simulink model "testFrame_PositionObserever"  (R2020b)
settings: Solver=FixedStepDiscrete  StartTime=0.0  StopTime=100  FixedStep=50e-6  RelTol=1e-3
undefined symbols (not defined in the file): d_q_Voltage_Limiter_sat_neg, d_q_Voltage_Limiter_sat_pos, Ts
libraries: mcbcontrolslib x4, pid_lib x2, simulink x1
settings Model: DataDictionary=MotorControl.sldd  NumberOfSteps=10  Creator=unix  LastModifiedBy=unix
settings DebuggingCC: IntegerOverflowMsg=error  ParameterUnderflowMsg=error  IntegerSaturationMsg=error

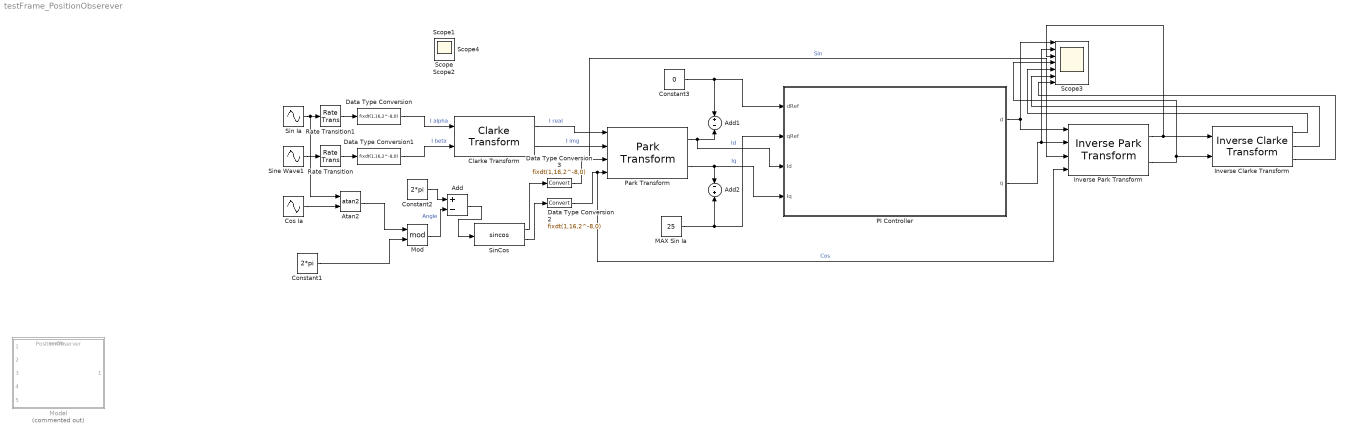
== system testFrame_PositionObserever ==
  Add : Sum  Inputs=+-
  Add1 : Sum  Inputs=+-  OutDataTypeStr=Inherit: Inherit via back propagation
  Add2 : Sum  Inputs=-+
  Atan2 : Trigonometry  Operator=atan2
  Clarke Transform : mcbcontrolslib/Clarke Transform  VariantControl=Variant2
  Constant1 : Constant  Value=2*pi  OutDataTypeStr=Inherit: Inherit via back propagation
  Constant2 : Constant  Value=2*pi  OutDataTypeStr=Inherit: Inherit via back propagation
  Constant3 : Constant  Value=0  OutDataTypeStr=int8
  Cos Ia : Sin  Amplitude=25  Frequency=100  Phase=pi/2  SampleTime=0
  Data Type Conversion{,1..3} (4 alike) : DataTypeConversion  OutDataTypeStr=fixdt(1,16,2^-8,0)
  Inverse Clarke Transform : mcbcontrolslib/Inverse Clarke Transform
      settings: SourceProductBaseCode=MT
  Inverse Park Transform : mcbcontrolslib/Inverse Park Transform  AxisAlignment=D-axis
  MAX Sin Ia : Constant  Value=25  OutDataTypeStr=Inherit: Inherit via back propagation
  Mod : Math  Operator=mod  SaturateOnIntegerOverflow=on
  Model : ModelReference  Commented=on  ModelNameDialog=PositionObserver.slx  ModelReferenceVersion=3.3  EnablePortName=Enable  EnablePortStatesWhenEnabling=reset
  PI Controller : Subsystem
  Park Transform : mcbcontrolslib/Park Transform  AxisAlignment=D-axis
      settings: SourceProductBaseCode=MT
  Rate Transition : RateTransition  OutPortSampleTime=250e-6
  Rate Transition1 : RateTransition  OutPortSampleTime=250e-6
  Scope3 : Scope  NumInputPorts=7
  Sin Ia : Sin  Amplitude=25  Frequency=100  SampleTime=0
  SinCos : Trigonometry  Operator=sincos
  Sine Wave1 : Sin  Amplitude=25  Frequency=100  Phase=(2*pi)/3  SampleTime=0
  Scope{,1..2,4} (4 alike) : Scope
  wires:
  SinCos/2 -> Data Type Conversion2/1
  SinCos/1 -> Data Type Conversion3/1
  Sin Ia/1 -> Atan2/1, Rate Transition1/1
  Sine Wave1/1 -> Rate Transition/1
  Clarke Transform/1 -> Park Transform/1  "I real"
  Clarke Transform/2 -> Park Transform/2  "I img"
  Constant1/1 -> Mod/2
  Park Transform/1 -> Add1/2, PI Controller/3(Id)  "Id"
  Park Transform/2 -> Add2/1, PI Controller/4(Iq)  "Iq"
  Data Type Conversion/1 -> Clarke Transform/1  "I alpha"
  Data Type Conversion1/1 -> Clarke Transform/2  "I beta"
  Mod/1 -> Add/2  "Angle"
  Data Type Conversion2/1 -> Inverse Park Transform/4, Park Transform/4  "Cos"
  Data Type Conversion3/1 -> Inverse Park Transform/3, Park Transform/3  "Sin"
  Rate Transition/1 -> Data Type Conversion1/1
  Rate Transition1/1 -> Data Type Conversion/1
  Constant2/1 -> Add/1
  Add/1 -> SinCos/1
  Constant3/1 -> Add1/1, PI Controller/1(dRef)
  MAX Sin Ia/1 -> Add2/2, PI Controller/2(qRef)
  PI Controller/1(d) -> Inverse Park Transform/1, Scope3/1
  PI Controller/2(q) -> Inverse Park Transform/2, Scope3/2
  Cos Ia/1 -> Atan2/2
  Atan2/1 -> Mod/1
  Inverse Park Transform/1 -> Inverse Clarke Transform/1, Scope3/3
  Inverse Park Transform/2 -> Inverse Clarke Transform/2, Scope3/4
  Inverse Clarke Transform/1 -> Scope3/5
  Inverse Clarke Transform/2 -> Scope3/6
  Inverse Clarke Transform/3 -> Scope3/7

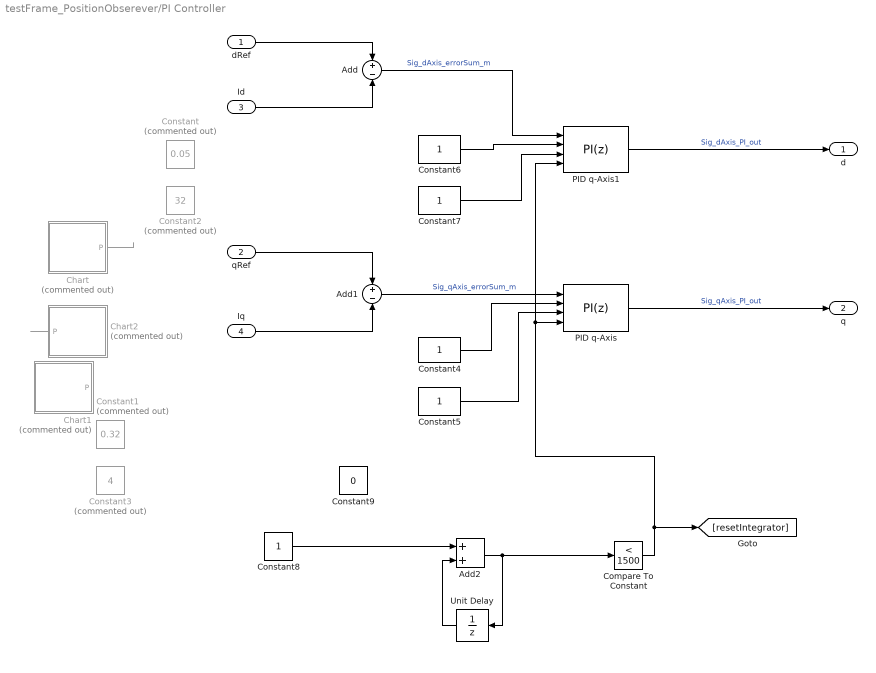
== system testFrame_PositionObserever/PI Controller ==
  dRef : Inport
  qRef : Inport  Port=2
  Id : Inport  Port=3
  Iq : Inport  Port=4
  Add : Sum  Inputs=+|-
  Add1 : Sum  Inputs=+|-
  Add2 : Sum
  Chart : Stateflow chart  Commented=on  TreatAsAtomicUnit=on  SystemSampleTime=1000*Ts
  Chart1 : Stateflow chart  Commented=on  TreatAsAtomicUnit=on  SystemSampleTime=2000*Ts
  Chart2 : Stateflow chart  Commented=on  TreatAsAtomicUnit=on  SystemSampleTime=100000*Ts
  Compare To Constant : simulink/Logic and Bit Operations/Compare To Constant  relop=<  const=1500  OutDataTypeStr=boolean
  Constant : Constant  Commented=on  Value=0.05  OutDataTypeStr=fixdt(1,16,2^-7,0)
  Constant1 : Constant  Commented=on  Value=0.32  OutDataTypeStr=fixdt(1,8,2^-7,0)
  Constant2 : Constant  Commented=on  Value=32  OutDataTypeStr=fixdt(1,8,2^-1,0)
  Constant3 : Constant  Commented=on  Value=4  OutDataTypeStr=fixdt(1,8,2^-1,0)
  Constant{4..7} (4 alike) : Constant  OutDataTypeStr=fixdt(1,16,2^-5,0)
  Constant8 : Constant
  Constant9 : Constant  Value=0  OutDataTypeStr=boolean
  PID q-Axis : pid_lib/PID Controller  Controller=PI  Form=Parallel  TimeDomain=Discrete-time  UseExternalTs=off  SampleTime=-1  IntegratorMethod=Forward Euler  FilterMethod=Forward Euler  ControllerParametersSource=external  P=0  I=0  D=0  UseFilter=on  N=100  TunerSelectOption=Transfer Function Based (PID Tuner App)  InitialConditionSource=internal  InitialConditionForIntegrator=0  InitialConditionForFilter=0  DifferentiatorICPrevScaledInput=0  ExternalReset=level  TrackingMode=off  Kt=1  LimitOutput=on  SatLimitsSource=internal  UpperSaturationLimit=d_q_Voltage_Limiter_sat_pos  LowerSaturationLimit=d_q_Voltage_Limiter_sat_neg  LinearizeAsGain=off  AntiWindupMode=clamping  Kb=10  PGainOutDataTypeStr=fixdt(1,16,2^-8,0)  PProdOutDataTypeStr=fixdt(1,16,2^-8,0)  POutMin=[]  POutMax=[]  IGainOutDataTypeStr=fixdt(1,16,2^-8,0)  IProdOutDataTypeStr=fixdt(1,16,2^-8,0)  IOutMin=[]  IOutMax=[]  DOutMin=[]  DOutMax=[]  NOutMin=[]  NOutMax=[]  SumOutDataTypeStr=fixdt(1,16,2^-8,0)  SumOutMin=[]  SumOutMax=[]  SaturationOutMin=[]  SaturationOutMax=[]  PParamMin=[]  PParamMax=[]  IParamMin=[]  IParamMax=[]  DParamMin=[]  DParamMax=[]  NParamMin=[]  NParamMax=[]  KbParamMin=[]  KbParamMax=[]  KtParamMin=[]  KtParamMax=[]  KbOutMin=[]  KbOutMax=[]  KtOutMin=[]  KtOutMax=[]  IntegratorOutDataTypeStr=fixdt(1,16,2^-8,0)  IntegratorOutMin=[]  IntegratorOutMax=[]  FilterOutMin=[]  FilterOutMax=[]  SumI1OutMin=[]  SumI1OutMax=[]  SumI2OutMin=[]  SumI2OutMax=[]  SumI3OutMin=[]  SumI3OutMax=[]  SumI4OutMin=[]  SumI4OutMax=[]  SumDOutMin=[]  SumDOutMax=[]  SumAccumDataTypeStr=fixdt(1,16,2^-8,0)  DifferentiatorOutMin=[]  DifferentiatorOutMax=[]  FilterDiffOutCoefMin=[]  FilterDiffOutCoefMax=[]  ReciprocalOutMin=[]  ReciprocalOutMax=[]  SumDenOutMin=[]  SumDenOutMax=[]  SumNumOutMin=[]  SumNumOutMax=[]  DivideOutMin=[]  DivideOutMax=[]  UdiffTsProdOutMin=[]  UdiffTsProdOutMax=[]  NTsProdOutMin=[]  NTsProdOutMax=[]  UintegralTsProdOutMin=[]  UintegralTsProdOutMax=[]  UngainTsProdOutMin=[]  UngainTsProdOutMax=[]  IntegratorContinuousStateAttributes=''  IntegratorStateMustResolveToSignalObject=off  IntegratorRTWStateStorageClass=Auto  FilterContinuousStateAttributes=''  FilterStateMustResolveToSignalObject=off  FilterRTWStateStorageClass=Auto  ParallelPVariant=ExternalParameters  IdealPVariant=Disabled  IVariant=ExternalParameters  DVariant=Disabled  IntegratorVariant=Discrete  SatVariant=Enabled  AWVariant=DiscClampingParallel  PCopyVariant=Disabled  TRVariant=Disabled  FdbkBlocksVariant=Forward  IdealPFdbkVariant=Disabled  SatFdbkVariant=Disabled  DerivativeFilterVariant=Disabled  NVariant=Disabled  NCopyVariant=Disabled_SignalSpec  FilterICVariant=Disabled  IntegratorICVariant=InternalICs  ExternalResetVariant=ExternalReset  TRSumVariant=Passthrough  SumFdbkVariant=Disabled  SumVariant=Sum_PI  TsampFilterVariant=InternalTs  TsampNgainVariant=Passthrough  TsampIntegralVariant=Passthrough  ExternalSaturationOutDataTypeStr=Inherit: Same as second input
  PID q-Axis1 : pid_lib/PID Controller  Controller=PI  Form=Parallel  TimeDomain=Discrete-time  UseExternalTs=off  SampleTime=-1  IntegratorMethod=Forward Euler  FilterMethod=Forward Euler  ControllerParametersSource=external  P=0  I=0  D=0  UseFilter=on  N=100  TunerSelectOption=Transfer Function Based (PID Tuner App)  ZeroCross=off  InitialConditionSource=internal  InitialConditionForIntegrator=0  InitialConditionForFilter=0  DifferentiatorICPrevScaledInput=0  ExternalReset=level  TrackingMode=off  Kt=1  LimitOutput=on  SatLimitsSource=internal  UpperSaturationLimit=d_q_Voltage_Limiter_sat_pos  LowerSaturationLimit=d_q_Voltage_Limiter_sat_neg  LinearizeAsGain=off  AntiWindupMode=clamping  Kb=10  PGainOutDataTypeStr=fixdt(1,16,2^-8,0)  PProdOutDataTypeStr=fixdt(1,16,2^-8,0)  POutMin=[]  POutMax=[]  IGainOutDataTypeStr=fixdt(1,16,2^-8,0)  IProdOutDataTypeStr=fixdt(1,16,2^-8,0)  IOutMin=[]  IOutMax=[]  DOutMin=[]  DOutMax=[]  NOutMin=[]  NOutMax=[]  SumOutDataTypeStr=fixdt(1,16,2^-8,0)  SumOutMin=[]  SumOutMax=[]  SaturationOutMin=[]  SaturationOutMax=[]  PParamMin=[]  PParamMax=[]  IParamMin=[]  IParamMax=[]  DParamMin=[]  DParamMax=[]  NParamMin=[]  NParamMax=[]  KbParamMin=[]  KbParamMax=[]  KtParamMin=[]  KtParamMax=[]  KbOutMin=[]  KbOutMax=[]  KtOutMin=[]  KtOutMax=[]  IntegratorOutDataTypeStr=fixdt(1,16,2^-8,0)  IntegratorOutMin=[]  IntegratorOutMax=[]  FilterOutMin=[]  FilterOutMax=[]  SumI1OutMin=[]  SumI1OutMax=[]  SumI2OutMin=[]  SumI2OutMax=[]  SumI3OutMin=[]  SumI3OutMax=[]  SumI4OutMin=[]  SumI4OutMax=[]  SumDOutMin=[]  SumDOutMax=[]  SumAccumDataTypeStr=fixdt(1,16,2^-8,0)  DifferentiatorOutMin=[]  DifferentiatorOutMax=[]  FilterDiffOutCoefMin=[]  FilterDiffOutCoefMax=[]  ReciprocalOutMin=[]  ReciprocalOutMax=[]  SumDenOutMin=[]  SumDenOutMax=[]  SumNumOutMin=[]  SumNumOutMax=[]  DivideOutMin=[]  DivideOutMax=[]  UdiffTsProdOutMin=[]  UdiffTsProdOutMax=[]  NTsProdOutMin=[]  NTsProdOutMax=[]  UintegralTsProdOutMin=[]  UintegralTsProdOutMax=[]  UngainTsProdOutMin=[]  UngainTsProdOutMax=[]  IntegratorContinuousStateAttributes=''  IntegratorStateMustResolveToSignalObject=off  IntegratorRTWStateStorageClass=Auto  FilterContinuousStateAttributes=''  FilterStateMustResolveToSignalObject=off  FilterRTWStateStorageClass=Auto  ParallelPVariant=ExternalParameters  IdealPVariant=Disabled  IVariant=ExternalParameters  DVariant=Disabled  IntegratorVariant=Discrete  SatVariant=Enabled  AWVariant=DiscClampingParallel  PCopyVariant=Disabled  TRVariant=Disabled  FdbkBlocksVariant=Forward  IdealPFdbkVariant=Disabled  SatFdbkVariant=Disabled  DerivativeFilterVariant=Disabled  NVariant=Disabled  NCopyVariant=Disabled_SignalSpec  FilterICVariant=Disabled  IntegratorICVariant=InternalICs  ExternalResetVariant=ExternalReset  TRSumVariant=Passthrough  SumFdbkVariant=Disabled  SumVariant=Sum_PI  TsampFilterVariant=InternalTs  TsampNgainVariant=Passthrough  TsampIntegralVariant=Passthrough  ExternalSaturationOutDataTypeStr=Inherit: Same as second input
  Unit Delay : UnitDelay  SampleTime=-1  HasFrameUpgradeWarning=on
  d : Outport
  q : Outport  Port=2
  wires:
  dRef/1 -> Add/1
  qRef/1 -> Add1/1
  Iq/1 -> Add1/2
  PID q-Axis/1 -> q/1  "Sig_qAxis_PI_out"
  PID q-Axis1/1 -> d/1  "Sig_dAxis_PI_out"
  Id/1 -> Add/2
  Add1/1 -> PID q-Axis/1  "Sig_qAxis_errorSum_m"
  Chart/1(P) -> ?
  Chart2/1(P) -> ?
  Constant5/1 -> PID q-Axis/3
  Constant4/1 -> PID q-Axis/2
  Add/1 -> PID q-Axis1/1  "Sig_dAxis_errorSum_m"
  Constant6/1 -> PID q-Axis1/2
  Constant7/1 -> PID q-Axis1/3
  Constant8/1 -> Add2/1
  Add2/1 -> Unit Delay/1, Compare To Constant/1
  Unit Delay/1 -> Add2/2
  Compare To Constant/1 -> [resetIntegrator], PID q-Axis1/4, PID q-Axis/4

== stateflow chart testFrame_PositionObserever/PI Controller/Chart1 ==
  (default) -> (junction 6) : /* P Value ++ */
  (junction 6) -> (junction 19) [order 1] : [P==0]{P=0.00;}
  (junction 6) -> (junction 17) [order 2]
  (junction 19) -> (junction 17)
  (junction 17) -> (junction 24) [order 2]
  (junction 17) -> (junction 8) [order 1] : {P+=0.1;}
  (junction 8) -> (junction 11) [order 2] : [P<=5]
  (junction 11) -> (junction 13)
  (junction 8) -> (junction 9) [order 1] : [P>5]{P=5;}
  (junction 9) -> (junction 13)
  data: P output double

== stateflow chart testFrame_PositionObserever/PI Controller/Chart ==
  (default) -> (junction 6) : /* P Value ++ */
  (junction 6) -> (junction 8) : {P+=0.001;}
  (junction 8) -> (junction 11) [order 2] : [P<=0]
  (junction 11) -> (junction 13)
  (junction 8) -> (junction 9) [order 1] : [P>0]{P=0.02;}
  (junction 9) -> (junction 13)
  data: P output double

== stateflow chart testFrame_PositionObserever/PI Controller/Chart2 ==
  (default) -> (junction 6) : /* P Value ++ */
  (junction 6) -> (junction 8) : {P+=1;}
  (junction 8) -> (junction 11) [order 2] : [P<=0]
  (junction 11) -> (junction 13)
  (junction 8) -> (junction 9) [order 1] : [P>0]{P=4;}
  (junction 9) -> (junction 13)
  data: P output double
